simulink model "Derivativeee"  (R2024a)
settings: Solver=VariableStepAuto  StartTime=0.0  StopTime=10.0  RelTol=1e-3
settings Model: Creator=mingyangpan

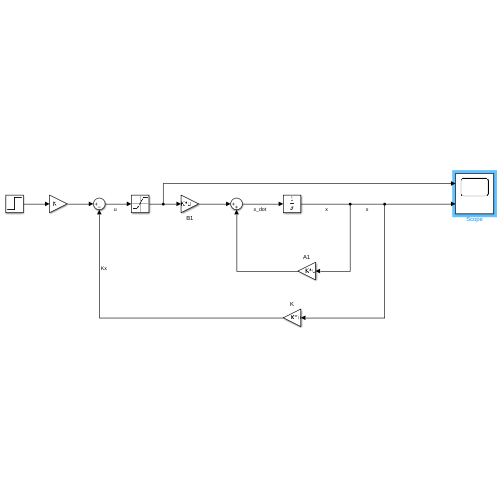
[thumbnail: Simulink's stored preview of the top-level diagram]
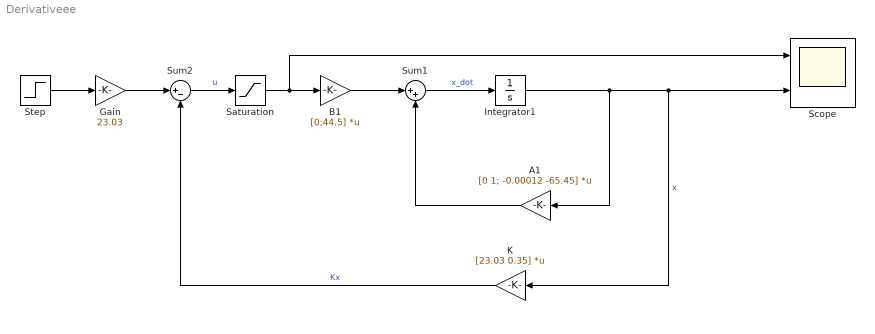
== system Derivativeee ==
  A1 : Gain  Gain=[0 1; -0.00012 -65.45]  Multiplication=Matrix(K*u)
  B1 : Gain  Gain=[0;44.5]  Multiplication=Matrix(K*u)
  Gain : Gain  Gain=23.03
  Integrator1 : Integrator
  K : Gain  Gain=[23.03 0.35]  Multiplication=Matrix(K*u)
  Saturation : Saturate  UpperLimit=300  LowerLimit=-300
  Scope : Scope  NumInputPorts=2
  Step : Step  Time=0.945  After=400  SampleTime=0
  Sum1 : Sum  Inputs=|++
  Sum2 : Sum  Inputs=|+-
  wires:
  B1/1 -> Sum1/1
  Saturation/1 -> Scope/1, B1/1
  Sum1/1 -> Integrator1/1  "x_dot"
  Integrator1/1 -> K/1, Scope/2, A1/1  "x"
  Sum2/1 -> Saturation/1  "u"
  A1/1 -> Sum1/2
  K/1 -> Sum2/2  "Kx"
  Gain/1 -> Sum2/1
  Step/1 -> Gain/1
